simulink model "CC_Three_point_guidance_law"  (R2024b)
settings: Solver=FixedStepAuto  StartTime=0.0  StopTime=50  FixedStep=0.01  RelTol=1e-3
settings Model: Creator=Acer  LastModifiedBy=Acer
settings DataIOCC: ReturnWorkspaceOutputs=off

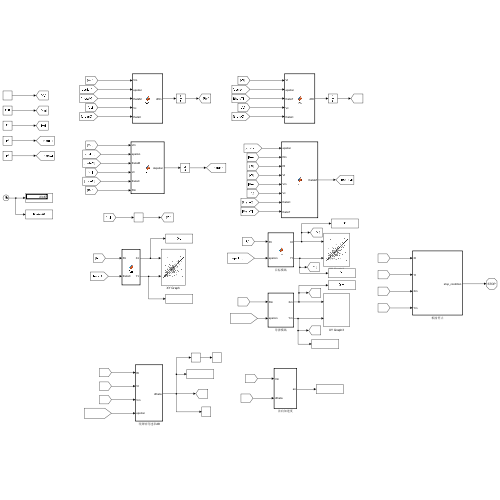
[thumbnail: Simulink's stored preview of the top-level diagram]
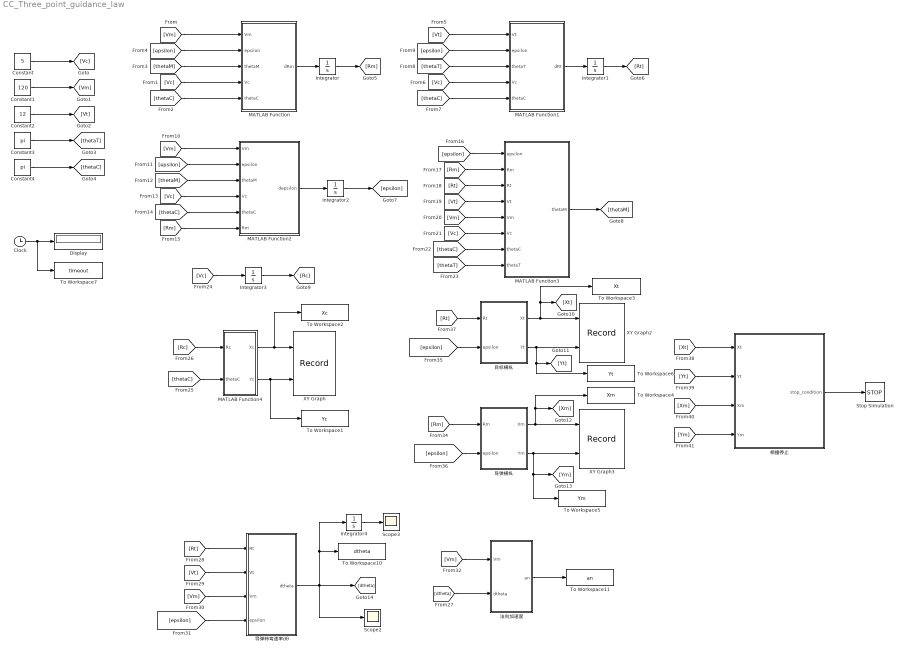
== system CC_Three_point_guidance_law ==
  Clock : Clock
  Constant : Constant  Value=5
  Constant1 : Constant  Value=120
  Constant2 : Constant  Value=12
  Constant3 : Constant  Value=pi
  Constant4 : Constant  Value=pi
  Display : Display
  Integrator : Integrator  InitialCondition=50
  Integrator1 : Integrator  InitialCondition=3000
  Integrator2 : Integrator  InitialCondition=70 * pi / 180
  Integrator3 : Integrator
  Integrator4 : Integrator  InitialCondition=70 * pi / 180
  MATLAB Function : MATLAB Function  TreatAsAtomicUnit=on
  MATLAB Function1 : MATLAB Function  TreatAsAtomicUnit=on
  MATLAB Function2 : MATLAB Function  TreatAsAtomicUnit=on
  MATLAB Function3 : MATLAB Function  TreatAsAtomicUnit=on
  MATLAB Function4 : MATLAB Function  TreatAsAtomicUnit=on
  Scope2 : Scope
  Scope3 : Scope
  Stop Simulation : Stop
  To Workspace1 : ToWorkspace  VariableName=Yc  SaveFormat=Timeseries  SampleTime=-1
  To Workspace10 : ToWorkspace  VariableName=dtheta  SaveFormat=Timeseries  SampleTime=-1
  To Workspace11 : ToWorkspace  VariableName=an  SaveFormat=Timeseries  SampleTime=-1
  To Workspace2 : ToWorkspace  VariableName=Xc  SaveFormat=Timeseries  SampleTime=-1
  To Workspace3 : ToWorkspace  VariableName=Xt  SaveFormat=Timeseries  SampleTime=-1
  To Workspace4 : ToWorkspace  VariableName=Xm  SaveFormat=Timeseries  SampleTime=-1
  To Workspace5 : ToWorkspace  VariableName=Ym  SaveFormat=Timeseries  SampleTime=-1
  To Workspace6 : ToWorkspace  VariableName=Yt  SaveFormat=Timeseries  SampleTime=-1
  To Workspace7 : ToWorkspace  VariableName=timeout  SaveFormat=Timeseries  SampleTime=-1
  XY Graph : Record  FileSettingsInternal="{\"entries\":[{\"content\":{\"excelSettings\":{\"content\":{},\"type\":\"Streamout.ExcelSettings\"}},\"type\":\"Streamout.FileSettingStorage\",\"uuid\":\"\"}],\"packageUris\":[\"http:\\/\\/schema.mathworks.com\\/mf0\\/streamout_blocks\\/R2020a\"],\"version\":\"1.0\"}"  Layout=[1 1]  SignalsInternal="{\"entries\":[{\"content\":{\"signals\":[{\"content\":{\"blockPath\":[],\"dimensions\":[1],\"domain\":\"\",\"lineColor\":\"#a2142f\",\"plots\":[ 1 ],\"port\":1,\"sid\":[\"\"],\"signalID\":1,\"signalName\":\"MATLAB Function4:1\"},\"type\":\"RecordBlkView.Signal\",\"uuid\":\"\"},{\"content\":{\"blockPath\":[],\"dimensions\":[1],\"domain\":\"\",\"lineColor\":\"#139fff\",\"plots\":[ 1 ],\"port\":2,\"sid\":[\"\"],\"signalID\":2,\"signalName\":\"MATLAB Function4:2\"},\"type\":\"RecordBlkView.Signal\",\"uuid\":\"\"}]},\"type\":\"RecordBlkView.InputSignals\",\"uuid\":\"\"}],\"packageUris\":[\"http:\\/\\/schema.mathworks.com\\/mf0\\/streamout_blocks\\/R2020a\"],\"version\":\"1.0\"}"  VisualizationBindings="{\"xyplotplugin\":{\"info\":[{\"series\":[{\"bindingParametersList\":[{\"parameter\":\"X-Axis\",\"signalID\":1,\"signalName\":\"MATLAB Function4:1\"},{\"parameter\":\"Y-Axis\",\"signalID\":2,\"signalName\":\"MATLAB Function4:2\"}],\"seriesID\":0}],\"subplotID\":1}]}}"  CompatibilityTag=XY
  XY Graph2 : Record  FileSettingsInternal="{\"entries\":[{\"content\":{\"excelSettings\":{\"content\":{},\"type\":\"Streamout.ExcelSettings\"}},\"type\":\"Streamout.FileSettingStorage\",\"uuid\":\"\"}],\"packageUris\":[\"http:\\/\\/schema.mathworks.com\\/mf0\\/streamout_blocks\\/R2020a\"],\"version\":\"1.0\"}"  Layout=[1 1]  SignalsInternal="{\"entries\":[{\"content\":{\"signals\":[{\"content\":{\"blockPath\":[],\"dimensions\":[1],\"domain\":\"\",\"lineColor\":\"#a2142f\",\"plots\":[ 1 ],\"port\":1,\"sid\":[\"\"],\"signalID\":1,\"signalName\":\"目标横纵:1\"},\"type\":\"RecordBlkView.Signal\",\"uuid\":\"\"},{\"content\":{\"blockPath\":[],\"dimensions\":[1],\"domain\":\"\",\"lineColor\":\"#139fff\",\"plots\":[ 1 ],\"port\":2,\"sid\":[\"\"],\"signalID\":2,\"signalName\":\"目标横纵:2\"},\"type\":\"RecordBlkView.Signal\",\"uuid\":\"\"}]},\"type\":\"RecordBlkView.InputSignals\",\"uuid\":\"\"}],\"packageUris\":[\"http:\\/\\/schema.mathworks.com\\/mf0\\/streamout_blocks\\/R2020a\"],\"version\":\"1.0\"}"  VisualizationBindings="{\"xyplotplugin\":{\"info\":[{\"series\":[{\"bindingParametersList\":[{\"parameter\":\"X-Axis\",\"signalID\":1,\"signalName\":\"目标横纵:1\"},{\"parameter\":\"Y-Axis\",\"signalID\":2,\"signalName\":\"目标横纵:2\"}],\"seriesID\":0}],\"subplotID\":1}]}}"  CompatibilityTag=XY
  XY Graph3 : Record  FileSettingsInternal="{\"entries\":[{\"content\":{\"excelSettings\":{\"content\":{},\"type\":\"Streamout.ExcelSettings\"}},\"type\":\"Streamout.FileSettingStorage\",\"uuid\":\"\"}],\"packageUris\":[\"http:\\/\\/schema.mathworks.com\\/mf0\\/streamout_blocks\\/R2020a\"],\"version\":\"1.0\"}"  Layout=[1 1]  SignalsInternal="{\"entries\":[{\"content\":{\"signals\":[{\"content\":{\"blockPath\":[],\"dimensions\":[1],\"domain\":\"\",\"lineColor\":\"#a2142f\",\"plots\":[ 1 ],\"port\":1,\"sid\":[\"\"],\"signalID\":1,\"signalName\":\"导弹横纵:1\"},\"type\":\"RecordBlkView.Signal\",\"uuid\":\"\"},{\"content\":{\"blockPath\":[],\"dimensions\":[1],\"domain\":\"\",\"lineColor\":\"#139fff\",\"plots\":[ 1 ],\"port\":2,\"sid\":[\"\"],\"signalID\":2,\"signalName\":\"导弹横纵:2\"},\"type\":\"RecordBlkView.Signal\",\"uuid\":\"\"}]},\"type\":\"RecordBlkView.InputSignals\",\"uuid\":\"\"}],\"packageUris\":[\"http:\\/\\/schema.mathworks.com\\/mf0\\/streamout_blocks\\/R2020a\"],\"version\":\"1.0\"}"  VisualizationBindings="{\"xyplotplugin\":{\"info\":[{\"series\":[{\"bindingParametersList\":[{\"parameter\":\"X-Axis\",\"signalID\":1,\"signalName\":\"导弹横纵:1\"},{\"parameter\":\"Y-Axis\",\"signalID\":2,\"signalName\":\"导弹横纵:2\"}],\"seriesID\":0}],\"subplotID\":1}]}}"  CompatibilityTag=XY
  导弹横纵 : MATLAB Function  TreatAsAtomicUnit=on
  导弹转弯速率dθ : MATLAB Function  TreatAsAtomicUnit=on
  法向加速度 : MATLAB Function  TreatAsAtomicUnit=on
  目标横纵 : MATLAB Function  TreatAsAtomicUnit=on
  相撞停止 : MATLAB Function  TreatAsAtomicUnit=on
  wires:
  Constant2/1 -> [Vt]
  Constant1/1 -> [Vm]
  Constant/1 -> [Vc]
  Constant3/1 -> [thetaT]
  Constant4/1 -> [thetaC]
  [Vm] -> MATLAB Function/1(Vm)
  [epsilon] -> MATLAB Function/2(epsilon)
  [thetaM] -> MATLAB Function/3(thetaM)
  [Vc] -> MATLAB Function/4(Vc)
  [thetaC] -> MATLAB Function/5(thetaC)
  MATLAB Function/1(dRm) -> Integrator/1
  Integrator/1 -> [Rm]
  Integrator1/1 -> [Rt]
  MATLAB Function1/1(dRt) -> Integrator1/1
  [thetaC] -> MATLAB Function1/5(thetaC)
  [Vc] -> MATLAB Function1/4(Vc)
  [thetaT] -> MATLAB Function1/3(thetaT)
  [epsilon] -> MATLAB Function1/2(epsilon)
  [Vt] -> MATLAB Function1/1(Vt)
  [Vm] -> MATLAB Function2/1(Vm)
  [epsilon] -> MATLAB Function2/2(epsilon)
  [thetaM] -> MATLAB Function2/3(thetaM)
  [Vc] -> MATLAB Function2/4(Vc)
  [thetaC] -> MATLAB Function2/5(thetaC)
  [Rm] -> MATLAB Function2/6(Rm)
  MATLAB Function2/1(depsilon) -> Integrator2/1
  Integrator2/1 -> [epsilon]
  [epsilon] -> MATLAB Function3/1(epsilon)
  [Rm] -> MATLAB Function3/2(Rm)
  [Vt] -> MATLAB Function3/4(Vt)
  [Rt] -> MATLAB Function3/3(Rt)
  [Vm] -> MATLAB Function3/5(Vm)
  [Vc] -> MATLAB Function3/6(Vc)
  [thetaC] -> MATLAB Function3/7(thetaC)
  [thetaT] -> MATLAB Function3/8(thetaT)
  MATLAB Function3/1(thetaM) -> [thetaM]
  [Vc] -> Integrator3/1
  Integrator3/1 -> [Rc]
  [thetaC] -> MATLAB Function4/2(thetaC)
  [Rc] -> MATLAB Function4/1(Rc)
  MATLAB Function4/1(Xc) -> To Workspace2/1, XY Graph/1
  MATLAB Function4/2(Yc) -> To Workspace1/1, XY Graph/2
  导弹横纵/1(Xm) -> To Workspace4/1, [Xm], XY Graph3/1
  [Rm] -> 导弹横纵/1(Rm)
  目标横纵/2(Yt) -> To Workspace6/1, [Yt], XY Graph2/2
  目标横纵/1(Xt) -> To Workspace3/1, [Xt], XY Graph2/1
  [epsilon] -> 目标横纵/2(epsilon)
  [epsilon] -> 导弹横纵/2(epsilon)
  [Rt] -> 目标横纵/1(Rt)
  导弹横纵/2(Ym) -> To Workspace5/1, [Ym], XY Graph3/2
  [Yt] -> 相撞停止/2(Yt)
  相撞停止/1(stop_condition) -> Stop Simulation/1
  [Xm] -> 相撞停止/3(Xm)
  [Xt] -> 相撞停止/1(Xt)
  [Ym] -> 相撞停止/4(Ym)
  Clock/1 -> To Workspace7/1, Display/1
  法向加速度/1(an) -> To Workspace11/1
  [dtheta] -> 法向加速度/2(dtheta)
  Integrator4/1 -> Scope3/1
  [Rt] -> 导弹转弯速率dθ/1(Rt)
  [Vm] -> 法向加速度/1(Vm)
  [epsilon] -> 导弹转弯速率dθ/4(epsilon)
  [Vt] -> 导弹转弯速率dθ/2(Vt)
  导弹转弯速率dθ/1(dtheta) -> Integrator4/1, To Workspace10/1, [dtheta], Scope2/1
  [Vm] -> 导弹转弯速率dθ/3(Vm)

== matlab function CC_Three_point_guidance_law/相撞停止 ==
  data: Xt input; stop_condition output; Yt input; Xm input; Ym input
function stop_condition = distance_check(Xt, Yt, Xm, Ym)
    
    distance = sqrt((Xt - Xm)^2 + (Yt - Ym)^2);
    stop_condition = distance < 1;
    
end

== matlab function CC_Three_point_guidance_law/MATLAB Function1 ==
  data: Vt input; dRt output; epsilon input; thetaT input; Vc input; thetaC input
function dRt = fcn(Vt, epsilon, thetaT, Vc, thetaC)
    dRt = Vt * cos(epsilon - thetaT) - Vc * cos(epsilon - thetaC);
end

== matlab function CC_Three_point_guidance_law/MATLAB Function ==
  data: Vm input; dRm output; epsilon input; thetaM input; Vc input; thetaC input
function dRm = fcn(Vm, epsilon, thetaM, Vc, thetaC)
    dRm = Vm * cos(epsilon - thetaM) - Vc * cos(epsilon - thetaC);
end

== matlab function CC_Three_point_guidance_law/MATLAB Function2 ==
  data: Vm input; depsilon output; epsilon input; thetaM input; Vc input; thetaC input; Rm input
function depsilon = fcn(Vm, epsilon, thetaM, Vc, thetaC, Rm)
    depsilon = ((-Vm) * sin(epsilon - thetaM) + Vc * sin(epsilon - thetaC)) / Rm;
end

== matlab function CC_Three_point_guidance_law/MATLAB Function3 ==
  data: epsilon input; thetaM output; Rm input; Rt input; Vt input; Vm input; Vc input; thetaC input; thetaT input
function thetaM = fcn(epsilon , Rm, Rt, Vt, Vm, Vc, thetaC, thetaT)
    thetaM = epsilon - asin((Rm / Rt) * ((Vt / Vm) * sin(epsilon - thetaT) - (Vc / Vm) * sin(epsilon - thetaC)) + (Vc / Vm) * sin(epsilon - thetaC));
end

== matlab function CC_Three_point_guidance_law/MATLAB Function4 ==
  data: Rc input; Xc output; thetaC input; Yc output
function [Xc, Yc] = fcn(Rc, thetaC)

Xc = Rc * cos(thetaC);
Yc = Rc * sin(thetaC);
end

== matlab function CC_Three_point_guidance_law/导弹转弯速率dθ ==
  data: Rt input; Vt input; dtheta output; Vm input; epsilon input
function dtheta = fcn(Rt, Vt, Vm, epsilon)
    p = Vm / Vt;    
    H = Rt * sin(epsilon);
    dtheta = (2 * Vt * ((sin(epsilon))^2) / H) * (1 + cos(epsilon) / sqrt(p^2 - ((sin(epsilon))^2)));
end

== matlab function CC_Three_point_guidance_law/法向加速度 ==
  data: Vm input; an output; dtheta input
function an = fcn(Vm, dtheta)
    an = Vm * dtheta;
end

== matlab function CC_Three_point_guidance_law/目标横纵 ==
  data: Rt input; Xt output; epsilon input; Yt output
function [Xt, Yt] = fcn(Rt, epsilon)

Xt = Rt * cos(epsilon);
Yt = Rt * sin(epsilon);

== matlab function CC_Three_point_guidance_law/导弹横纵 ==
  data: Rm input; Xm output; epsilon input; Ym output
function [Xm, Ym] = fcn(Rm, epsilon)

Xm = Rm * cos(epsilon);
Ym = Rm * sin(epsilon);
